simulink model "MRAC_actuator_fault_tolerant"  (R2015b)
settings: Solver=VariableStepAuto  StartTime=0.0  StopTime=100  RelTol=1e-3
settings Model: Creator=admin  LastModifiedBy=admin

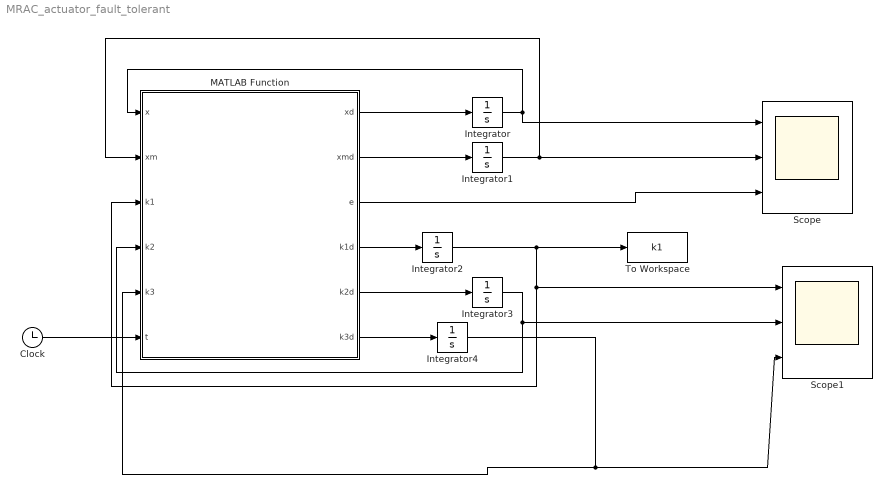
== system MRAC_actuator_fault_tolerant ==
  Clock : Clock
  Integrator : Integrator  InitialCondition=[0;0]
  Integrator1 : Integrator  InitialCondition=[0;0]
  Integrator2 : Integrator  InitialCondition=[0 0;0 0]
  Integrator3 : Integrator  InitialCondition=[0 0]
  Integrator4 : Integrator  InitialCondition=[0 0]
  MATLAB Function : MATLAB Function  TreatAsAtomicUnit=on
  Scope : Scope  NumInputPorts=3
  Scope1 : Scope  NumInputPorts=3
  To Workspace : ToWorkspace  VariableName=k1  SaveFormat=Timeseries  SampleTime=-1
  wires:
  MATLAB Function/1(xd) -> Integrator/1
  MATLAB Function/2(xmd) -> Integrator1/1
  MATLAB Function/5(k2d) -> Integrator3/1
  Integrator/1 -> Scope/1, MATLAB Function/1(x)
  Integrator1/1 -> Scope/2, MATLAB Function/2(xm)
  Integrator3/1 -> MATLAB Function/4(k2), Scope1/2
  MATLAB Function/3(e) -> Scope/3
  Clock/1 -> MATLAB Function/6(t)
  MATLAB Function/6(k3d) -> Integrator4/1
  Integrator4/1 -> MATLAB Function/5(k3), Scope1/3
  MATLAB Function/4(k1d) -> Integrator2/1
  Integrator2/1 -> To Workspace/1, MATLAB Function/3(k1), Scope1/1

== matlab function MRAC_actuator_fault_tolerant/MATLAB Function ==
  data: x input; xm input; xd output; k1 input; k2 input; k3 input; xmd output; e output; k1d output; k2d output; t input; k3d output
function [xd,xmd,e,k1d,k2d,k3d] = fcn(x,xm,k1,k2,k3,t)

if(t<40)
     sigma=diag([0,0]);
else
     sigma=diag([1,0]);
end
    
e=x-xm;
r=(1-exp(-t));

% Controller
%sigma=diag([0,0]);
v=k1'*x+k2*r+k3;
u_bar1=0;
u_bar2=0;
u_bar=[u_bar1; u_bar2];
u=v+sigma*(u_bar-v);

%system model(which is unknown in real cases, we only have information about the state only which is measurable)
A=[-1 1; 0 -2];
B=[1 (2/3);1.5 1];
xd=A*x+B*u;

ks2_star=[2;3];

%Reference model
Am=[-2 1; 0 -3];
Bm=[2 ;3];

xmd=Am*xm+Bm*r;
% Controller parameter update law
P=[1/4 1/20;1/20 11/60];
gamma1_1=[1 1;1 1];
gamma1_2=[1 1;1 1];
gamma2_1=1;
gamma2_2=1;
gamma3_1=1;
gamma3_2=1;
%gamma1=[gamma1_1;gamma1_2]; % By changing the gains we can only change the transient state,
gamma2=[gamma2_1;gamma2_2]; % steady state performance will be same
gamma3=[gamma3_1;gamma3_2]; % check for any other error if error is not zero
k1d_1=-gamma1_1*x*e'*P*Bm*sign(ks2_star(1));
k2d_1=-gamma2(1)*r*e'*P*Bm*sign(ks2_star(1));
k3d_1=-gamma3(1)*e'*P*Bm*sign(ks2_star(1));
k1d_2=-gamma1_2*x*e'*P*Bm*sign(ks2_star(2));
k2d_2=-gamma2(2)*r*e'*P*Bm*sign(ks2_star(2));
k3d_2=-gamma3(2)*e'*P*Bm*sign(ks2_star(2));
k1d=[k1d_1 k1d_2];
k2d=[k2d_1;k2d_2];
k3d=[k3d_1;k3d_2];
